simulink model "VehicleSteering_sim"  (Simulink 8.3)
settings: Solver=ode45  SolverMode=SingleTasking  StartTime=0.0  StopTime=10.0  RelTol=1e-3
values from neighbouring files (symbols this model uses):
  A = [0 v0;0 0]    [Example_VehicleSteering_Integral_action.m]    (also in Example_VehicleSteering_LQR.m; Example_VehicleSteering_SS_control.m)
  B = [a*v0/b v0/b]'    [Example_VehicleSteering_Integral_action.m]    (also in Example_VehicleSteering_LQR.m; Example_VehicleSteering_SS_control.m)
  C = eye(2)    [Example_VehicleSteering_Integral_action.m]    (also in Example_VehicleSteering_LQR.m; Example_VehicleSteering_SS_control.m)
  D = [0 0]'    [Example_VehicleSteering_Integral_action.m]    (also in Example_VehicleSteering_LQR.m; Example_VehicleSteering_SS_control.m)
  K = [b*wn^2/v0^2 (2*zeta*wn*b/v0-a*b*wn^2/v0^2)]    [Example_VehicleSteering_SS_control.m]
  kr = -1/([1 0]* (A-B*K)*B)^(-1)    [Example_VehicleSteering_LQR.m]    (also in Example_VehicleSteering_SS_control.m = 0.444444444444)
settings Model: Creator=jofr  LastModifiedBy=rodralez  CovMetricSettings=dwe  CovHtmlReporting=off  covSaveCumulativeToWorkspaceVar=off  CovSaveSingleToWorkspaceVar=off  CovExternalEMLEnable=on  CovSFcnEnable=on
settings DataIOCC: LimitDataPoints=off  SaveFormat=StructureWithTime  SignalLoggingSaveFormat=Dataset
settings DebuggingCC: UnderspecifiedInitializationDetection=Simplified  MergeDetectMultiDrivingBlocksExec=error  SolverPrmCheckMsg=none  FrameProcessingCompatibilityMsg=error  StateNameClashWarn=none  SFUnexpectedBacktrackingDiag=error  SFNoUnconditionalDefaultTransitionDiag=error
settings HardwareCC: ProdBitPerPointer=64  ProdLargestAtomicFloat=Float  ProdIntDivRoundTo=Zero  ProdEndianess=LittleEndian  ProdHWDeviceType=Specified
settings ModelReferenceCC: PropagateSignalLabelsOutOfModel=on
settings GRTTargetCC: TargetLangStandard=C99 (ISO)  CombineOutputUpdateFcns=on  GRTInterface=off

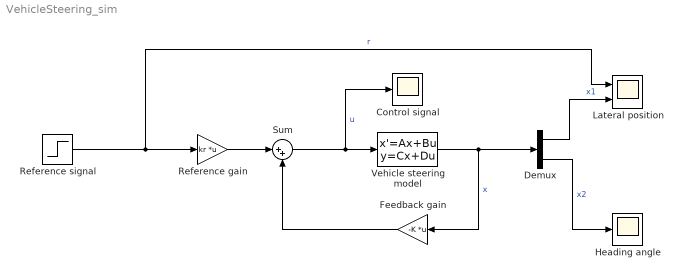
== system VehicleSteering_sim ==
  Control signal : Scope
      settings: TimeRange=auto  MaxDataPoints=5000  SaveName=u  YMin=-0.0077  YMax=0.03172  SampleTime=-1  DataFormat=Array
  Demux : Demux  Outputs=2
  Feedback gain : Gain  Gain=-K  Multiplication=Matrix(K*u)
  Heading angle : Scope
      settings: TimeRange=auto  MaxDataPoints=5000  SaveName=x2  YMin=-0.00383  YMax=0.03449  SampleTime=-1  DataFormat=Array
  Lateral position : Scope  NumInputPorts=2
      settings: TimeRange=auto  MaxDataPoints=5000  SaveName=x1  YMin=-0.125~-5  YMax=1.125~5  SampleTime=-1  DataFormat=Structure
  Reference gain : Gain  Gain=kr  Multiplication=Matrix(K*u)
  "Reference signal " : Step  SampleTime=0
  Sum : Sum  Inputs=|++
  Vehicle steering model : StateSpace  A=A  B=B  C=C  D=D  X0=0
  wires:
  Vehicle steering model/1 -> Demux/1, Feedback gain/1  "x"
  Sum/1 -> Control signal/1, Vehicle steering model/1  "u"
  Feedback gain/1 -> Sum/2
  Reference gain/1 -> Sum/1
  Demux/2 -> Heading angle/1  "x2"
  "Reference signal "/1 -> Lateral position/1, Reference gain/1  "r"
  Demux/1 -> Lateral position/2  "x1"
